simulink model "FSK_m70"  (Simulink 7.6)
settings: Solver=ode45  StartTime=0.0  StopTime=sim_t  RelTol=1e-3
undefined symbols (not defined in the file): A1f, A2f, BSTf, F1f, F2f, PZf, STf
libraries: commrandsrc2 x1, simulink x1, commsynccomp2 x1
settings Model: Creator=usuario  LastModifiedBy=cocheca
settings OptimizationCC: InitFltsAndDblsToZero=on
settings DebuggingCC: SaveWithParameterizedLinksMsg=none  SignalResolutionControl=TryResolveAllWithWarning  MultiTaskDSMMsg=warning  MultiTaskCondExecSysMsg=none  StrictBusMsg=Warning
settings RTWCC: IncludeERTFirstTime=on
settings GRTTargetCC: TargetFcnLib=ansi_tfl_tmw.mat

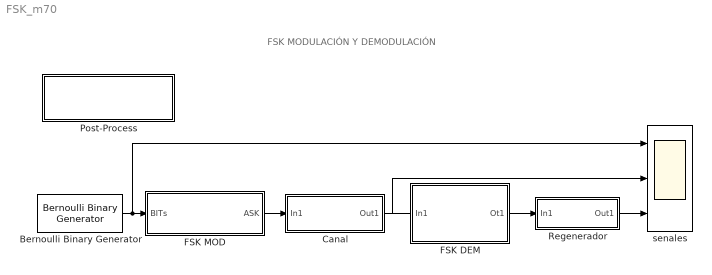
== system FSK_m70 ==
  note: FSK MODULACIÓN Y DEMODULACIÓN
  Bernoulli Binary Generator : commrandsrc2/Bernoulli Binary Generator  DialogController=commDDGCreate  DialogControllerArgs=DataTag0  SystemSampleTime=-1  P=PZf  seed=61  Ts=BSTf  frameBased=off  sampPerFrame=1  orient=off  outDataType=double
  Canal : Subsystem
  FSK DEM : Subsystem
  FSK MOD : Subsystem
  Post-Process : Subsystem  mask{sim_t=50, BSTf=3, F1f=6000, A1f=1, F2f=12000, A2f=1}
      mask prompts: sim_t "Sim Time [100]"; BSTf "Source Sample Time"; F1f "Freq. Sine 1 [8K]"; A1f "Amp. Sine 1 [1]"; F2f "Freq. Sine 2 [12K]"; A2f "Amp. Sine 2 [1]"
      mask init:
      | %sim_t = 100; %simulation time
      | %BSTf = 5; % source sample time
      | PZf = .3; % probability of zero
      | 
      | %STf = 1/100; % sample time
      | %A1f = 1; % amplitude sine 1 - mod.
      | %A2f = 1; % amplitude sine 2 - mod.
      | %F1f = 2*pi*8; % Freg Sine 1
      | %F2f = 2*pi*12; % Freg Sine 2
      | 
      | switch sim_t
      |     case 1
      |         sim_t = 25;
      |     case 2
      |         sim_t = 50;
      |     case 3
      |         sim_t = 100;
      |     case 4
      |         sim_t = 150;   
      | end
      | 
      | % Sample Time Source Configure
      | switch BSTf
      |     case 1
      |         BSTf = 3;
      |     case 2
      |         BSTf = 5;
      |     case 3
      |         BSTf = 8;
      |     case 4
      |         BSTf = 10;
      |     case 5
      |         BSTf = 12;        
      | end
      | 
      | switch F1f
      |     case 1
      |         F1f = 6000;
      |     case 2
      |         F1f = 8000;
      |     case 3
      |         F1f = 10000;
      |     case 4
      |         F1f = 16000;
      | end
      | 
      | switch F2f
      |     case 1
      |         F2f = 8000;
      |     case 2    
      |         F2f = 10000;
      |     case 3        
      |         F2f = 12000;
      |     case 4
      |         F2f = 16000;
      | end
      | 
      | STf=(1/BSTf*5/100);
      | F1f=2*pi*F1f/1000;
      | F2f=2*pi*F2f/1000;
      | 
      | assignin('base','sim_t', sim_t );
      | assignin('base','BSTf', BSTf );
      | assignin('base','PZf', PZf );
      | assignin('base','STf', STf );
      | assignin('base','A1f', A1f );
      | assignin('base','A2f', A2f );
      | assignin('base','F1f', F1f );
      | assignin('base','F2f', F2f );
      mask StyleString: popup(25|50|100|250),popup(3|5|8|10|12),popup(6000|8000|10000|16000),edit,popup(8000|10000|12000|16000),edit
      mask Display: disp('Sim Parameters')
  Regenerador : Subsystem
  senales : Scope  NumInputPorts=3
      settings: YMin=-0.5~-2~-0.5  YMax=1.5~2~1.5
  wires:
  Bernoulli Binary Generator/1 -> FSK MOD/1(BITs), senales/1
  FSK MOD/1(ASK) -> Canal/1(In1)
  FSK DEM/1(Ot1) -> Regenerador/1(In1)
  Canal/1(Out1) -> FSK DEM/1(In1), senales/2
  Regenerador/1(Out1) -> senales/3

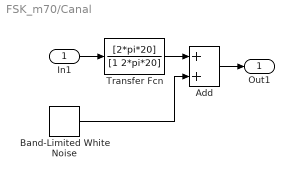
== system FSK_m70/Canal ==
  In1 : Inport
  Add : Sum
  Band-Limited White Noise : simulink/Sources/Band-Limited White Noise  SystemSampleTime=-1  Cov=[0.002]  Ts=1  seed=[23341]
  Transfer Fcn : TransferFcn  Numerator=[2*pi*20]  Denominator=[1 2*pi*20]
  Out1 : Outport
  wires:
  Transfer Fcn/1 -> Add/1
  Band-Limited White Noise/1 -> Add/2
  In1/1 -> Transfer Fcn/1
  Add/1 -> Out1/1

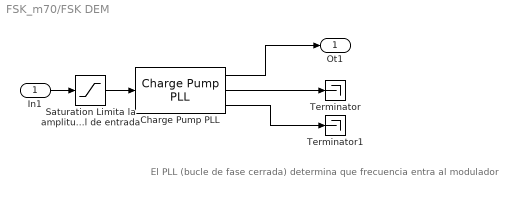
== system FSK_m70/FSK DEM ==
  note: El PLL (bucle de fase cerrada)
      | determina que frecuencia
      | entra al modulador
  In1 : Inport
  Charge Pump PLL : commsynccomp2/Charge Pump PLL  SystemSampleTime=-1  Fn=[2*pi*1]  Fd="[1   2*pi*1]"  Kvco=4  Fc=10  Ph=0  Ac=1
  Saturation Limita la amplitud de la señal de entrada : Saturate
  Terminator : Terminator
  Terminator1 : Terminator
  Ot1 : Outport
  wires:
  In1/1 -> Saturation Limita la amplitud de la señal de entrada/1
  Saturation Limita la amplitud de la señal de entrada/1 -> Charge Pump PLL/1
  Charge Pump PLL/1 -> Ot1/1
  Charge Pump PLL/2 -> Terminator/1
  Charge Pump PLL/3 -> Terminator1/1

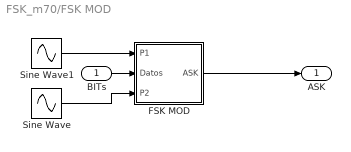
== system FSK_m70/FSK MOD ==
  BITs : Inport
  FSK MOD : Subsystem
  Sine Wave : Sin  Amplitude=A2f  Frequency=F2f  Samples=25  SampleTime=STf
  Sine Wave1 : Sin  Amplitude=A1f  Frequency=F1f  Samples=50  SampleTime=STf
  ASK : Outport
  wires:
  BITs/1 -> FSK MOD/2(Datos)
  FSK MOD/1(ASK) -> ASK/1
  Sine Wave1/1 -> FSK MOD/1(P1)
  Sine Wave/1 -> FSK MOD/3(P2)

== system FSK_m70/Post-Process ==

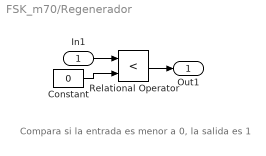
== system FSK_m70/Regenerador ==
  note: Compara si la entrada
      | es menor a 0, la salida es 1
  In1 : Inport
  Constant : Constant  Value=0
  Relational Operator : RelationalOperator  Operator=<  OutDataTypeStr=boolean
  Out1 : Outport
  wires:
  Relational Operator/1 -> Out1/1
  In1/1 -> Relational Operator/1
  Constant/1 -> Relational Operator/2

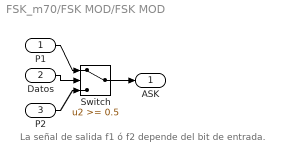
== system FSK_m70/FSK MOD/FSK MOD ==
  note: La señal de salida f1 ó f2
      | depende del bit de entrada.
  P1 : Inport
  Datos : Inport  Port=2
  P2 : Inport  Port=3
  Switch : Switch  Threshold=0.5
  ASK : Outport
  wires:
  P1/1 -> Switch/1
  Datos/1 -> Switch/2
  Switch/1 -> ASK/1
  P2/1 -> Switch/3
